simulink model "for_paper_CFDLMFAC"  (R2018b)
settings: Solver=ode4  StartTime=0.0  StopTime=30  FixedStep=0.00625  RelTol=1e-3
values from neighbouring files (symbols this model uses):
  CornerFreq = 1.570796    [Run_CFDLMFAC.m]
  initalAgl = 0    [Run_CFDLMFAC.m]
  PC_KI = 0.004068634    [Run_CFDLMFAC.m]
  PC_KK = 0.1099965    [Run_CFDLMFAC.m]
  PC_KP = 0.01882681    [Run_CFDLMFAC.m]
  PC_MaxPit = 1.570796    [Run_CFDLMFAC.m]
  PC_RefSpd = 122.9096    [Run_CFDLMFAC.m]
  R2D = 57.295780    (= 57.29578)    [Run_CFDLMFAC.m]
undefined symbols (not defined in the file or in its folder): OutList, strmatch
libraries: simulink x1, cstblocks x1
settings Model: Creator=lijia  LastModifiedBy=lijia

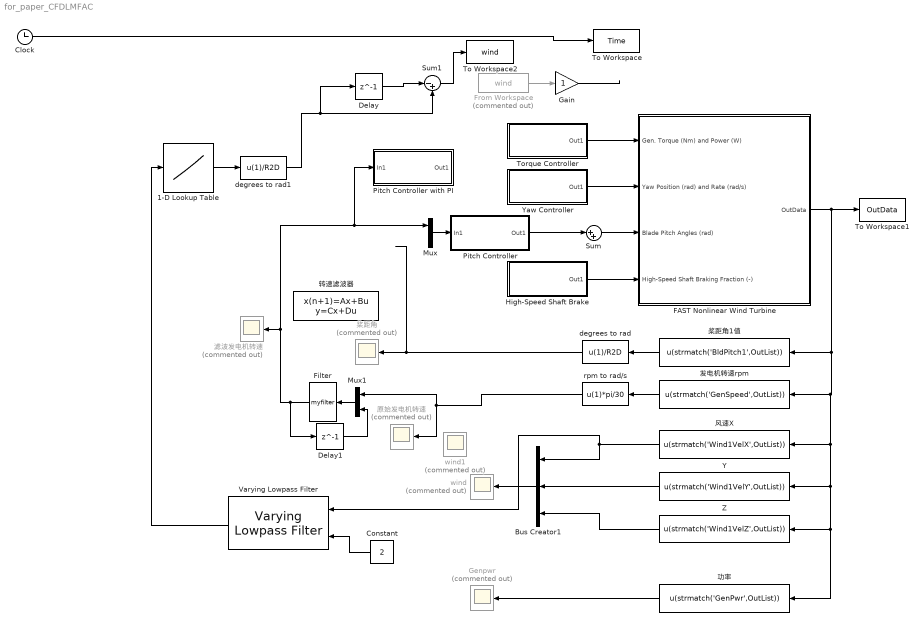
== system for_paper_CFDLMFAC ==
  1-D Lookup Table : Lookup_n-D  NumberOfTableDimensions=1  LookupTableObject=wind_deg  BreakpointsForDimension1=[11.4,12,13,14,15,16,17,18,19,20,21,22,23,24,25]  Table=[0,2.55,5.65,7.85,9.69,11.35,12.86,14.27,15.63,16.96,18.23,19.46,20.65,21.8,22.92]  InterpMethod=Cubic spline  ExtrapMethod=Clip  InternalRulePriority=Speed  OutMin=[0]  OutMax=[90]  RndMeth=Simplest  InputSameDT=on
  Bus Creator1 : BusCreator  Inputs=3
  Clock : Clock
  Constant : Constant  Value=2
  Delay : Delay  DelayLength=1
  Delay1 : Delay  DelayLength=1
  FAST Nonlinear Wind Turbine : Subsystem  mask(FAST Nonlinear Wind Turbine){}
      mask help: This block contains the FAST S-Function.
      mask init:
      | clear FAST_SFunc
  Filter : S-Function  FunctionName=myfilter  SFunctionDeploymentMode=off  EnableBusSupport=off
  From Workspace : FromWorkspace  Commented=on  VariableName=wind
  Gain : Gain
  Genpwr : Scope  Commented=on
  High-Speed Shaft Brake : Subsystem
  Mux : Mux  Inputs=2
  Mux1 : Mux  Inputs=2
  Pitch Controller : Subsystem
  Pitch Controller with PI : Subsystem
  Sum : Sum  Inputs=|++
  Sum1 : Sum  Inputs=|-+
  To Workspace : ToWorkspace  VariableName=Time  SampleTime=-1
  To Workspace1 : ToWorkspace  VariableName=OutData  SampleTime=-1
  To Workspace2 : ToWorkspace  VariableName=wind  SaveFormat=Timeseries  SampleTime=-1
  Torque Controller : Subsystem
  Varying Lowpass Filter : cstblocks/Linear Parameter Varying/Varying Lowpass Filter  N=2
      settings: SourceProductName=Control System Toolbox
  Y : Fcn  Expr=u(strmatch('Wind1VelY',OutList))
  Yaw Controller : Subsystem
  Z : Fcn  Expr=u(strmatch('Wind1VelZ',OutList))
  degrees to rad : Fcn  Expr=u(1)/R2D
  degrees to rad1 : Fcn  Expr=u(1)/R2D
  rpm to rad/s : Fcn  Expr=u(1)*pi/30
  wind : Scope  Commented=on
  wind1 : Scope  Commented=on
  功率 : Fcn  Expr=u(strmatch('GenPwr',OutList))
  原始发电机转速 : Scope  Commented=on
  发电机转速rpm : Fcn  Expr=u(strmatch('GenSpeed',OutList))
  桨距角 : Scope  Commented=on
  桨距角1值 : Fcn  Expr=u(strmatch('BldPitch1',OutList))
  滤波发电机转速 : Scope  Commented=on
  转速滤波器 : DiscreteStateSpace  A=exp(-(0.0063)*CornerFreq)  B=1-exp(-0.0063*CornerFreq)  C=exp(-0.0063*CornerFreq)  D=1-exp(-0.0063*CornerFreq)  SampleTime=-1
  风速X : Fcn  Expr=u(strmatch('Wind1VelX',OutList))
  wires:
  Sum/1 -> FAST Nonlinear Wind Turbine/3(Blade Pitch Angles (rad))
  High-Speed Shaft Brake/1(Out1) -> FAST Nonlinear Wind Turbine/4(High-Speed Shaft Braking Fraction (-))
  FAST Nonlinear Wind Turbine/1(OutData) -> Y/1, Z/1, 功率/1, 风速X/1, 发电机转速rpm/1, 桨距角1值/1, To Workspace1/1
  Yaw Controller/1(Out1) -> FAST Nonlinear Wind Turbine/2(Yaw Position (rad) and Rate (rad/s))
  Clock/1 -> To Workspace/1
  桨距角1值/1 -> degrees to rad/1
  Torque Controller/1(Out1) -> FAST Nonlinear Wind Turbine/1(Gen. Torque (Nm) and Power (W))
  degrees to rad/1 -> 桨距角/1
  功率/1 -> Genpwr/1
  Y/1 -> Bus Creator1/2
  Z/1 -> Bus Creator1/3
  Bus Creator1/1 -> wind/1
  发电机转速rpm/1 -> rpm to rad/s/1
  风速X/1 -> Varying Lowpass Filter/1, Bus Creator1/1
  rpm to rad/s/1 -> Mux1/1, 原始发电机转速/1
  Mux/1 -> Pitch Controller/1(In1)
  Varying Lowpass Filter/1 -> 1-D Lookup Table/1
  Constant/1 -> Varying Lowpass Filter/2
  1-D Lookup Table/1 -> degrees to rad1/1
  Delay/1 -> Sum1/1
  degrees to rad1/1 -> Sum1/2, Delay/1
  From Workspace/1 -> Gain/1
  Gain/1 -> ?
  Sum1/1 -> To Workspace2/1
  Pitch Controller/1(Out1) -> Sum/1
  Delay1/1 -> Mux1/2
  Mux1/1 -> Filter/1
  Filter/1 -> Delay1/1, 滤波发电机转速/1, Pitch Controller with PI/1(In1), Mux/1

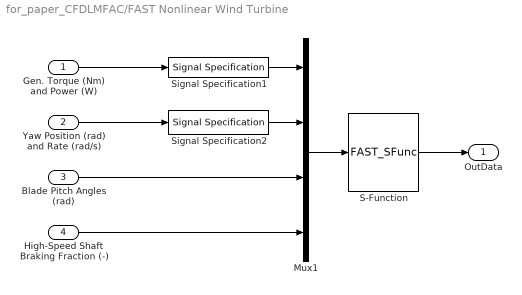
== system for_paper_CFDLMFAC/FAST Nonlinear Wind Turbine ==
  Gen. Torque (Nm) and Power (W) : Inport
  Yaw Position (rad) and Rate (rad/s) : Inport  Port=2
  Blade Pitch Angles (rad) : Inport  Port=3
  High-Speed Shaft Braking Fraction (-) : Inport  Port=4
  Mux1 : Mux
  S-Function : S-Function  FunctionName=FAST_SFunc  Parameters=FAST_InputFileName, TMax, 0  SFunctionDeploymentMode=off  EnableBusSupport=off
  Signal Specification1 : SignalSpecification  OutDataTypeStr=double  Dimensions=2
  Signal Specification2 : SignalSpecification  OutDataTypeStr=double  Dimensions=2
  OutData : Outport
  wires:
  Gen. Torque (Nm) and Power (W)/1 -> Signal Specification1/1
  S-Function/1 -> OutData/1
  Mux1/1 -> S-Function/1
  Blade Pitch Angles (rad)/1 -> Mux1/3
  Yaw Position (rad) and Rate (rad/s)/1 -> Signal Specification2/1
  Signal Specification1/1 -> Mux1/1
  Signal Specification2/1 -> Mux1/2
  High-Speed Shaft Braking Fraction (-)/1 -> Mux1/4

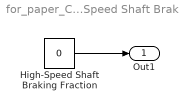
== system for_paper_CFDLMFAC/High-Speed Shaft Brake ==
  High-Speed Shaft Braking Fraction : Constant  Value=0
  Out1 : Outport
  wires:
  High-Speed Shaft Braking Fraction/1 -> Out1/1

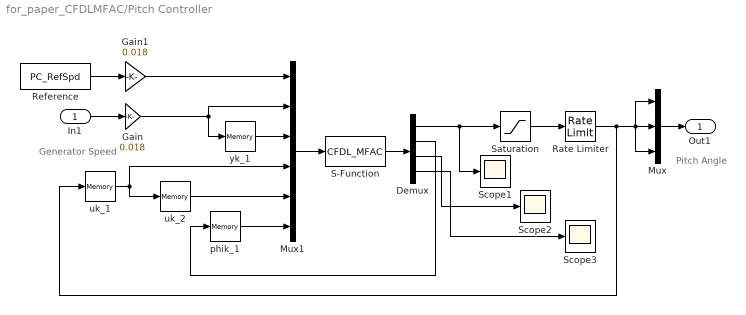
== system for_paper_CFDLMFAC/Pitch Controller ==
  note: Pitch Angle
  note: Generator Speed
  In1 : Inport
  Demux : Demux
  Gain : Gain  Gain=0.018
  Gain1 : Gain  Gain=0.018
  Mux : Mux  Inputs=3
  Mux1 : Mux  Inputs=6
  Rate Limiter : RateLimiter  RisingSlewLimit=0.1396263  FallingSlewLimit=-0.1396263  SampleTimeMode=inherited  InitialCondition=initalAgl
  Reference : Constant  Value=PC_RefSpd
  S-Function : S-Function  FunctionName=CFDL_MFAC  SFunctionDeploymentMode=off  EnableBusSupport=off
  Saturation : Saturate  UpperLimit=1.5708  LowerLimit=0
  Scope1 : Scope
  Scope2 : Scope
  Scope3 : Scope
  phik_1 : Memory  InitialCondition=-10
  uk_1 : Memory  InitialCondition=initalAgl
  uk_2 : Memory  InitialCondition=initalAgl
  yk_1 : Memory  InitialCondition=2.2
  Out1 : Outport
  wires:
  Mux/1 -> Out1/1
  Mux1/1 -> S-Function/1
  S-Function/1 -> Demux/1
  phik_1/1 -> Mux1/6
  Demux/2 -> phik_1/1
  Rate Limiter/1 -> Mux/3, Mux/2, Mux/1, uk_1/1
  In1/1 -> Gain/1
  Reference/1 -> Gain1/1
  Demux/3 -> Scope2/1
  yk_1/1 -> Mux1/3
  uk_2/1 -> Mux1/5
  Gain1/1 -> Mux1/1
  Saturation/1 -> Rate Limiter/1
  uk_1/1 -> Mux1/4, uk_2/1
  Gain/1 -> yk_1/1, Mux1/2
  Demux/4 -> Scope3/1
  Demux/1 -> Scope1/1, Saturation/1

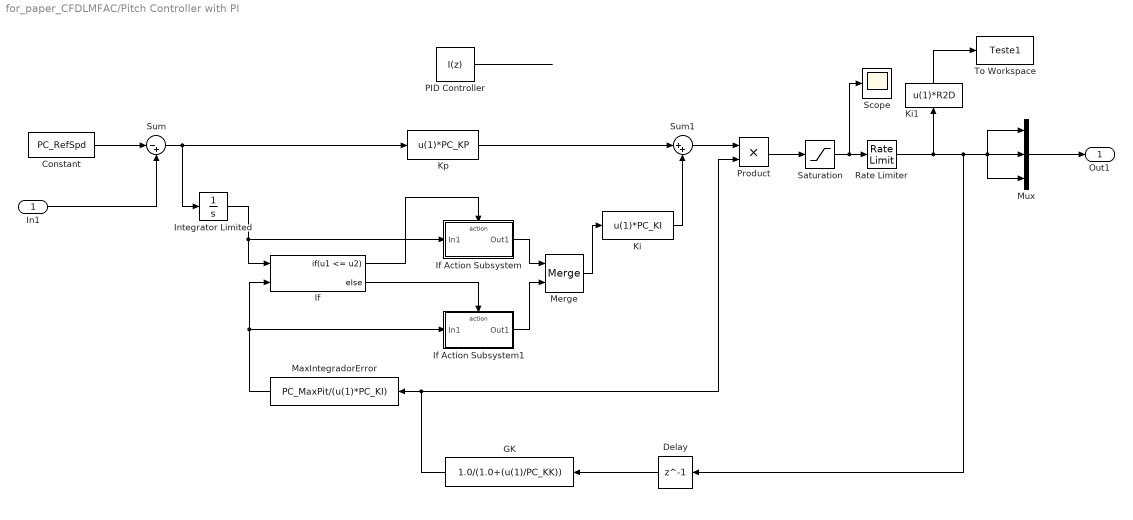
== system for_paper_CFDLMFAC/Pitch Controller with PI ==
  In1 : Inport
  Constant : Constant  Value=PC_RefSpd
  Delay : Delay  DelayLength=1  InitialCondition=0
  GK : Fcn  Expr=1.0/(1.0+(u(1)/PC_KK))
  If : If  NumInputs=2  IfExpression=u1 <= u2
  If Action Subsystem : Subsystem  TreatAsAtomicUnit=on
  If Action Subsystem1 : Subsystem  TreatAsAtomicUnit=on
  Integrator Limited : Integrator  LimitOutput=on  UpperSaturationLimit=1.57079/PC_KI  LowerSaturationLimit=0  IgnoreLimit=on
  Ki : Fcn  Expr=u(1)*PC_KI
  Ki1 : Fcn  Expr=u(1)*R2D
  Kp : Fcn  Expr=u(1)*PC_KP
  MaxIntegradorError : Fcn  Expr=PC_MaxPit/(u(1)*PC_KI)
  Merge : Merge
  Mux : Mux  Inputs=3
  PID Controller : simulink/Continuous/PID Controller  Controller=I  Form=Parallel  TimeDomain=Discrete-time  SampleTime=-1  IntegratorMethod=Forward Euler  FilterMethod=Forward Euler  ControllerParametersSource=internal  P=PC_KP  I=PC_KI  D=0.1  UseFilter=on  N=100  TunerSelectOption=Transfer Function Based (PID Tuner App)  InitialConditionSource=internal  InitialConditionForIntegrator=0  InitialConditionForFilter=0  DifferentiatorICPrevScaledInput=0  ExternalReset=none  TrackingMode=off  Kt=1  LimitOutput=off  UpperSaturationLimit=inf  LowerSaturationLimit=-inf  LinearizeAsGain=on  AntiWindupMode=none  Kb=1  POutMin=[]  POutMax=[]  IOutMin=[]  IOutMax=[]  DOutMin=[]  DOutMax=[]  NOutMin=[]  NOutMax=[]  SumOutMin=[]  SumOutMax=[]  SaturationOutMin=[]  SaturationOutMax=[]  PParamMin=[]  PParamMax=[]  IParamMin=[]  IParamMax=[]  DParamMin=[]  DParamMax=[]  NParamMin=[]  NParamMax=[]  KbParamMin=[]  KbParamMax=[]  KtParamMin=[]  KtParamMax=[]  KbOutMin=[]  KbOutMax=[]  KtOutMin=[]  KtOutMax=[]  IntegratorOutMin=[]  IntegratorOutMax=[]  FilterOutMin=[]  FilterOutMax=[]  SumI1OutMin=[]  SumI1OutMax=[]  SumI2OutMin=[]  SumI2OutMax=[]  SumI3OutMin=[]  SumI3OutMax=[]  SumI4OutMin=[]  SumI4OutMax=[]  SumDOutMin=[]  SumDOutMax=[]  DifferentiatorOutMin=[]  DifferentiatorOutMax=[]  FilterDiffOutCoefMin=[]  FilterDiffOutCoefMax=[]  ReciprocalOutMin=[]  ReciprocalOutMax=[]  SumDenOutMin=[]  SumDenOutMax=[]  SumNumOutMin=[]  SumNumOutMax=[]  DivideOutMin=[]  DivideOutMax=[]  IntegratorContinuousStateAttributes=''  IntegratorStateMustResolveToSignalObject=off  IntegratorRTWStateStorageClass=Auto  FilterContinuousStateAttributes=''  FilterStateMustResolveToSignalObject=off  FilterRTWStateStorageClass=Auto  ParallelPVariant=Disabled  IdealPVariant=Disabled  IVariant=InternalParameters  DVariant=Disabled  IntegratorVariant=Discrete  SatVariant=Disabled  AWVariant=Passthrough  PCopyVariant=Disabled  TRVariant=Disabled  FdbkBlocksVariant=Forward  IdealPFdbkVariant=Disabled  SatFdbkVariant=Disabled  DerivativeFilterVariant=Disabled  NVariant=Disabled  NCopyVariant=Disabled_SignalSpec  FilterICVariant=Disabled  IntegratorICVariant=InternalICs  ExternalResetVariant=Disabled  TRSumVariant=Passthrough  SumFdbkVariant=Disabled  SumVariant=Passthrough_I
  Product : Product
  Rate Limiter : RateLimiter  RisingSlewLimit=0.1396263  FallingSlewLimit=-0.1396263  SampleTimeMode=inherited
  Saturation : Saturate  UpperLimit=1.5708  LowerLimit=0
  Scope : Scope
  Sum : Sum  Inputs=|-+
  Sum1 : Sum  Inputs=|++
  To Workspace : ToWorkspace  VariableName=Teste1  SaveFormat=Timeseries  SampleTime=-1
  Out1 : Outport
  wires:
  Ki1/1 -> To Workspace/1
  Saturation/1 -> Rate Limiter/1, Scope/1
  GK/1 -> Product/2, MaxIntegradorError/1
  Delay/1 -> GK/1
  Sum1/1 -> Product/1
  Kp/1 -> Sum1/1
  Ki/1 -> Sum1/2
  Merge/1 -> Ki/1
  If Action Subsystem1/1(Out1) -> Merge/2
  If Action Subsystem/1(Out1) -> Merge/1
  MaxIntegradorError/1 -> If/2, If Action Subsystem1/1(In1)
  If/2 -> If Action Subsystem1/Action
  If/1 -> If Action Subsystem/Action
  Integrator Limited/1 -> If/1, If Action Subsystem/1(In1)
  In1/1 -> Sum/2
  Constant/1 -> Sum/1
  Product/1 -> Saturation/1
  Sum/1 -> Kp/1, Integrator Limited/1
  Mux/1 -> Out1/1
  Rate Limiter/1 -> Ki1/1, Mux/1, Mux/3, Mux/2, Delay/1
  PID Controller/1 -> ?

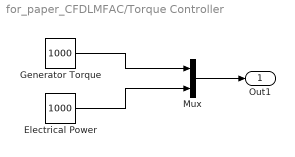
== system for_paper_CFDLMFAC/Torque Controller ==
  Electrical Power : Constant  Value=1000
  Generator Torque : Constant  Value=1000
  Mux : Mux  Inputs=2
  Out1 : Outport
  wires:
  Mux/1 -> Out1/1
  Generator Torque/1 -> Mux/1
  Electrical Power/1 -> Mux/2

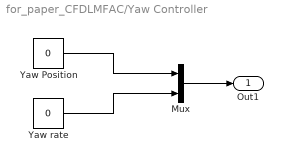
== system for_paper_CFDLMFAC/Yaw Controller ==
  Mux : Mux  Inputs=2
  Yaw Position : Constant  Value=0
  Yaw rate : Constant  Value=0
  Out1 : Outport
  wires:
  Mux/1 -> Out1/1
  Yaw Position/1 -> Mux/1
  Yaw rate/1 -> Mux/2

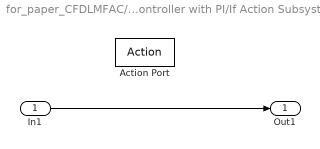
== system for_paper_CFDLMFAC/Pitch Controller with PI/If Action Subsystem ==
  In1 : Inport
  Action Port : ActionPort  ActionType=then
  Out1 : Outport
  wires:
  In1/1 -> Out1/1

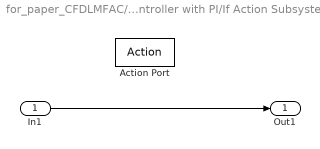
== system for_paper_CFDLMFAC/Pitch Controller with PI/If Action Subsystem1 ==
  In1 : Inport
  Action Port : ActionPort  ActionType=else
  Out1 : Outport
  wires:
  In1/1 -> Out1/1
